simulink model "algebraic_demo"  (Simulink 6.3)
settings: Solver=ode45  StartTime=0.0  StopTime=10.0  RelTol=1e-3
libraries: simulink x2
settings Model: LastModifiedBy=Ms1

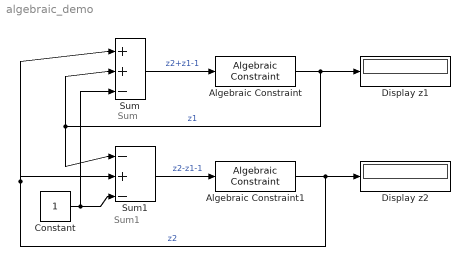
== system algebraic_demo ==
  note: Sum1
  note: Sum
  Algebraic Constraint : simulink/Math Operations/Algebraic Constraint  z0=0
  Algebraic Constraint1 : simulink/Math Operations/Algebraic Constraint  z0=0
  Constant : Constant
  Display z1 : Display
  Display z2 : Display
  Sum : Sum  Inputs=|++-  SaturateOnIntegerOverflow=on  InputSameDT=on
  Sum1 : Sum  Inputs=|-+-  SaturateOnIntegerOverflow=on  InputSameDT=on
  wires:
  Constant/1 -> Sum/3, Sum1/3
  Sum1/1 -> Algebraic Constraint1/1  "z2-z1-1"
  Sum/1 -> Algebraic Constraint/1  "z2+z1-1"
  Algebraic Constraint1/1 -> Display z2/1, Sum/1, Sum1/2  "z2"
  Algebraic Constraint/1 -> Display z1/1, Sum/2, Sum1/1  "z1"
